simulink model "Distribution_Fault_Model"  (R2025a)
settings: Solver=VariableStepAuto  StartTime=0.0  StopTime=1  RelTol=1e-3
undefined symbols (not defined in the file or in its folder): Angle, D1, Delta, Magnitude
libraries: spsThreePhasePISectionLineLib x8, spsThreePhaseVIMeasurementLib x5, spsThreePhaseTransformerTwoWindingsLib x5, spsCurrentMeasurementLib x4, spsThreePhaseSeriesRLCLoadLib x4, spsGroundLib x3, spsVoltageMeasurementLib x3, spsThreePhaseSourceLib x1, spsThreePhaseFaultLib x1, spsSeriesRLCBranchLib x1, spspowerguiLib x1
settings Model: Creator=19092  LastModifiedBy=19092

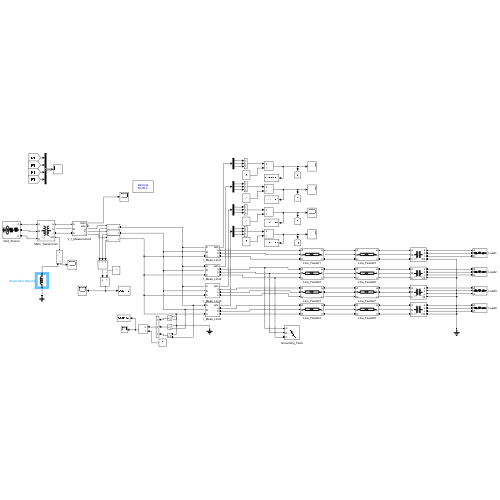
[thumbnail: Simulink's stored preview of the top-level diagram]
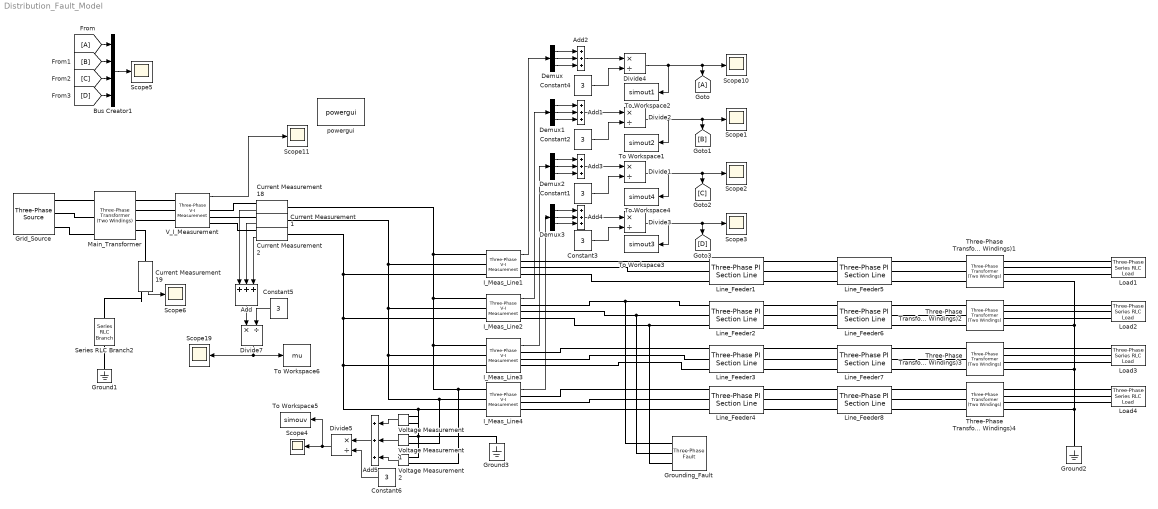
== system Distribution_Fault_Model ==
  Add{,1..5} (6 alike) : Sum  Inputs=+++
  Bus Creator1 : BusCreator  Inputs=4
  Constant{1..6} (6 alike) : Constant  Value=3
  Current Measurement{1..2,18..19} (4 alike) : spsCurrentMeasurementLib/Current Measurement  PhasorSimulation=off  OutputType=Magnitude-Angle  PSBequivalent=0
  Demux{,1..3} (4 alike) : Demux  Outputs=3
  Divide{1..5,7} (6 alike) : Product  Inputs=*/
  From : From
  Goto : Goto
  Grid_Source : spsThreePhaseSourceLib/Three-Phase Source  InternalConnection=Yg  VoltagePhases=off  Voltage=110e3  PhaseAngle=0  Voltage_phases=[25e3 25e3 25e3]/sqrt(3)  PhaseAngles_phases=[0 -120 +120]  Frequency=50  NonIdealSource=on  SpecifyImpedance=off  Resistance=0.8  Inductance=16.58e-3  ShortCircuitLevel=100e6  BaseVoltage=25e3  XRratio=7  BusType=swing  Pref=10e3  Qref=0  Prefabc=[10e3, 10e3, 10e3]  Qrefabc=[0, 0, 0]  Qmin=-inf  Qmax=inf
  Ground1 : spsGroundLib/Ground  LConnTagsString=a
  Ground2 : spsGroundLib/Ground  LConnTagsString=a
  Ground3 : spsGroundLib/Ground  LConnTagsString=a
  Grounding_Fault : spsThreePhaseFaultLib/Three-Phase Fault  InitialStates=0  FaultA=on  FaultB=off  FaultC=off  GroundFault=on  SwitchTimes=0.105  External=off  SwitchStatus=NaN  FaultResistance=100  GroundResistance=0.00000001  SnubberResistance=1e6  SnubberCapacitance=inf  Measurements=None
  I_Meas_Line{1..4} (4 alike) : spsThreePhaseVIMeasurementLib/Three-Phase V-I Measurement  VoltageMeasurement=no  SetLabelV=off  LabelV=Vabc  Vpu=off  VpuLL=off  CurrentMeasurement=yes  SetLabelI=off  LabelI=Iabc  Ipu=off  Pbase=100e6  Vbase=500e3  OutputType=Complex  PhasorSimulation=off  PSBequivalent=0
  Line_Feeder{1..4} (4 alike) : spsThreePhasePISectionLineLib/Three-Phase PI Section Line  LConnTagsString=a|b|c  RConnTagsString=A|B|C  Length=3  Frequency=50  Resistances=[0.27 2.7 ]  Inductances="[0.255e-3  1.109e-3]"  Capacitances=[0.376e-6 0.276e-6]
  Line_Feeder5 : spsThreePhasePISectionLineLib/Three-Phase PI Section Line  LConnTagsString=a|b|c  RConnTagsString=A|B|C  Length=15  Frequency=50  Resistances=[0.17 0.32 ]  Inductances="[1.017e-3  3.56e-3]"  Capacitances=[0.115e-6 0.006e-6]
  Line_Feeder6 : spsThreePhasePISectionLineLib/Three-Phase PI Section Line  LConnTagsString=a|b|c  RConnTagsString=A|B|C  Length=6  Frequency=50  Resistances=[0.27 2.7 ]  Inductances="[0.255e-3  1.109e-3]"  Capacitances=[0.376e-6 0.276e-6]
  Line_Feeder7 : spsThreePhasePISectionLineLib/Three-Phase PI Section Line  LConnTagsString=a|b|c  RConnTagsString=A|B|C  Length=6  Frequency=50  Resistances=[0.17 0.32 ]  Inductances="[ 1.017e-3  3.56e-3]"  Capacitances=[0.115e-6 0.006e-6]
  Line_Feeder8 : spsThreePhasePISectionLineLib/Three-Phase PI Section Line  LConnTagsString=a|b|c  RConnTagsString=A|B|C  Length=6  Frequency=50  Resistances=[0.17 0.32 ]  Inductances="[ 1.017e-3  3.56e-3]"  Capacitances=[0.115e-6 0.006e-6]
  Load{1..4} (4 alike) : spsThreePhaseSeriesRLCLoadLib/Three-Phase Series RLC Load  LConnTagsString=A|B|C  Configuration=Y (grounded)  NominalVoltage=380  Vabc=[1e3 1e3 1e3]  Vabcp=[1e3 1e3 1e3]  NominalFrequency=50  UnbalancedPower=off  ActivePower=0.8e5  InductivePower=0.5e5  CapacitivePower=0.2e5  Pabc=[10e3 9e3 11e3]  QLabc=[100 90 110]  QCabc=[100 90 110]  Pabcp=[10e3 9e3 11e3]  QLabcp=[100 90 110]  QCabcp=[100 90 110]  Measurements=None  LoadType=constant Z
  Main_Transformer : spsThreePhaseTransformerTwoWindingsLib/Three-Phase Transformer (Two Windings)  Winding1Connection=Yg  Winding2Connection=Yn  CoreType=Three single-phase transformers  SetSaturation=off  Hysteresis=off  DataFile='hysteresis'  SetInitialFlux=off  Measurements=None  UNITS=SI  NominalPower=[ 30e6 , 50 ]  Winding1=[1.1e+05 97.607 0.039558]  Winding2=[11000 0.0080667 3.2693e-06]  Rm=2.4402e+07  Lm=247.24  L0=0.64192  Saturation=[0 0;0.53443 343.07;222.68 434.55]  InitialFluxes=[228.71 -228.71 200.12]  BreakLoop=off  DiscreteSolver=Trapezoidal iterative  DataType=on  TransfoNumber=1
  Scope{1..6,10..11,19} (9 alike) : Scope
      Scope1 settings: ActiveDisplayYMinimum=-457.04126923383052  ActiveDisplayYMaximum=338.42605854849973  DataLoggingVariableName=ZAOlingxudianliu
      Scope10 settings: ActiveDisplayYMinimum=-5.367403011968813  ActiveDisplayYMaximum=5.1815718746200288  DataLoggingVariableName=ZAOlingxudianliu1
      Scope11 settings: ActiveDisplayYMinimum=-30411.319643702398  ActiveDisplayYMaximum=29803.514177511406
      Scope19 settings: ActiveDisplayYMinimum=-66.79577978771502  ActiveDisplayYMaximum=84.3725838120956  DataLoggingVariableName=ScopeData5
      Scope2 settings: ActiveDisplayYMinimum=-2.9181062576325916  ActiveDisplayYMaximum=2.3384047230485843  DataLoggingVariableName=ZAOlingxudianliu2
      Scope3 settings: ActiveDisplayYMinimum=-3.7719258239086075  ActiveDisplayYMaximum=3.3149529318803035  DataLoggingVariableName=ZAOlingxudianliu3
      Scope4 settings: ActiveDisplayYMinimum=-11360.33274  ActiveDisplayYMaximum=9549.66393  DataLoggingVariableName=ScopeData2
      Scope5 settings: ActiveDisplayYMinimum=-55.84943  ActiveDisplayYMaximum=52.05941
      Scope6 settings: ActiveDisplayYMinimum=-133.27899753443887  ActiveDisplayYMaximum=70.5276469261506  DataLoggingVariableName=ScopeData3
  Series RLC Branch2 : spsSeriesRLCBranchLib/Series RLC Branch  LConnTagsString=__new0  RConnTagsString=__new0  BranchType=L  Resistance=100  Inductance=0.6  SetiL0=off  InitialCurrent=0  Capacitance=1e-6  Setx0=off  InitialVoltage=0  Measurements=None
  Three-Phase Transformer (Two Windings){1..4} (4 alike) : spsThreePhaseTransformerTwoWindingsLib/Three-Phase Transformer (Two Windings)  Winding1Connection=Delta (D1)  Winding2Connection=Yn  CoreType=Three single-phase transformers  SetSaturation=off  Hysteresis=off  DataFile='hysteresis'  SetInitialFlux=off  Measurements=None  UNITS=SI  NominalPower=[5e6 , 50 ]  Winding1=[10e3 27.011 3.4392]  Winding2=[400 0.005 0.00063662]  Rm=6.7528e+06  Lm=21495  L0=0.5  Saturation=[0 0;0.10664 2292.3;44.435 2903.6]  InitialFluxes=[1528.2 -1528.2 1337.2]  BreakLoop=off  DiscreteSolver=Trapezoidal iterative  DataType=on  TransfoNumber=1
  To Workspace1 : ToWorkspace  VariableName=simout2  SaveFormat=Structure With Time  SampleTime=-1
  To Workspace2 : ToWorkspace  VariableName=simout1  SaveFormat=Structure With Time  SampleTime=-1
  To Workspace3 : ToWorkspace  VariableName=simout3  SaveFormat=Structure With Time  SampleTime=-1
  To Workspace4 : ToWorkspace  VariableName=simout4  SaveFormat=Structure With Time  SampleTime=-1
  To Workspace5 : ToWorkspace  VariableName=simouv  SaveFormat=Structure With Time  SampleTime=-1
  To Workspace6 : ToWorkspace  VariableName=mu  SaveFormat=Structure With Time  SampleTime=-1
  V_I_Measurement : spsThreePhaseVIMeasurementLib/Three-Phase V-I Measurement  VoltageMeasurement=phase-to-ground  SetLabelV=off  LabelV=Vabc  Vpu=off  VpuLL=off  CurrentMeasurement=yes  SetLabelI=off  LabelI=Iabc  Ipu=off  Pbase=100e6  Vbase=500e3  OutputType=Complex  PhasorSimulation=off  PSBequivalent=0
  Voltage Measurement : spsVoltageMeasurementLib/Voltage Measurement  PhasorSimulation=off  OutputType=Complex  PSBequivalent=0
  Voltage Measurement1 : spsVoltageMeasurementLib/Voltage Measurement  PhasorSimulation=off  OutputType=Complex  PSBequivalent=0
  Voltage Measurement2 : spsVoltageMeasurementLib/Voltage Measurement  PhasorSimulation=off  OutputType=Complex  PSBequivalent=0
  powergui : spspowerguiLib/powergui  Priority=1  SimulationMode=Discrete  SampleTime=50e-6  frequency=50  Iterations=50  frequencyindice=50  Pbase=100e6  ErrMax=1e-4  UnitsV=kV  UnitsW=MW  buscounter=0  FunctionMessages=off  echomessages=off  EnableUseOfTLC=off  CurrentSourceSwitches=off  DisableSnubberDevices=off  DisableRonSwitches=off  DisableVfSwitches=off  DisplayEquations=off  AutomaticDiscreteSolvers=off  SolverType=Tustin/Backward Euler (TBE)  Interpol=off  ExternalGateDelay=off  methode=off  Ts=100  x0status=blocks  SPID=on  SwTol=0  HookPort=off  NonlinearTolerance=1e-4  nMaxIteration=100  ContinueOnMaxIteration=off  RestoreLinks=warning  ResistiveCurrentMeasurement=off  Frange=[0:2:500]  Ylog=off  Xlog=on  ShowGrid=off  save=off  variable=ZData  structure=0  ZoomFFT=off  StartTime=0.0  cycles=1  DisplayStyle=1  fundamental=50  FreqAxis=off  MaxFrequency=1000  frequencyindicesteady=1  RmsSteady=1  display=off
  wires:
  V_I_Measurement/1 -> Scope11/1
  Current Measurement18/1 -> Add/1
  Current Measurement1/1 -> Add/2
  Current Measurement2/1 -> Add/3
  I_Meas_Line1/1 -> Demux/1
  I_Meas_Line2/1 -> Demux1/1
  I_Meas_Line4/1 -> Demux3/1
  Demux/1 -> Add2/1
  Demux/2 -> Add2/2
  Demux/3 -> Add2/3
  Demux1/1 -> Add1/1
  Demux1/2 -> Add1/2
  Demux1/3 -> Add1/3
  Demux2/1 -> Add3/1
  Demux2/2 -> Add3/2
  Demux2/3 -> Add3/3
  Demux3/1 -> Add4/1
  Demux3/2 -> Add4/2
  Demux3/3 -> Add4/3
  Add4/1 -> Divide3/1
  Constant3/1 -> Divide3/2
  Constant1/1 -> Divide1/2
  Add3/1 -> Divide1/1
  Constant2/1 -> Divide2/2
  Add1/1 -> Divide2/1
  Constant4/1 -> Divide4/2
  Add2/1 -> Divide4/1
  I_Meas_Line3/1 -> Demux2/1
  Divide3/1 -> [D], Scope3/1, To Workspace3/1
  Divide1/1 -> [C], Scope2/1, To Workspace4/1
  Divide2/1 -> [B], Scope1/1, To Workspace1/1
  Divide4/1 -> Goto/1, Scope10/1, To Workspace2/1
  [C] -> Bus Creator1/3
  [B] -> Bus Creator1/2
  From/1 -> Bus Creator1/1
  [D] -> Bus Creator1/4
  Bus Creator1/1 -> Scope5/1
  Current Measurement19/1 -> Scope6/1
  Constant5/1 -> Divide7/2
  Add/1 -> Divide7/1
  Divide7/1 -> Scope19/1, To Workspace6/1
  Constant6/1 -> Divide5/2
  Add5/1 -> Divide5/1
  Voltage Measurement/1 -> Add5/1
  Voltage Measurement1/1 -> Add5/2
  Voltage Measurement2/1 -> Add5/3
  Divide5/1 -> To Workspace5/1, Scope4/1
  connections:
  Grid_Source/RConn1 -- Main_Transformer/LConn1
  Grid_Source/RConn2 -- Main_Transformer/LConn2
  Grid_Source/RConn3 -- Main_Transformer/LConn3
  Main_Transformer/RConn1 -- V_I_Measurement/LConn1
  Main_Transformer/RConn2 -- V_I_Measurement/LConn2
  Main_Transformer/RConn3 -- V_I_Measurement/LConn3
  V_I_Measurement/RConn1 -- Current Measurement18/RConn1
  V_I_Measurement/RConn2 -- Current Measurement1/RConn1
  V_I_Measurement/RConn3 -- Current Measurement2/RConn1
  I_Meas_Line1/RConn2 -- Line_Feeder1/LConn2
  I_Meas_Line1/RConn3 -- Line_Feeder1/LConn3
  Line_Feeder1/LConn1 -- I_Meas_Line1/RConn1
  I_Meas_Line2/RConn1 -- Grounding_Fault/LConn1 -- Line_Feeder2/LConn1
  I_Meas_Line2/RConn2 -- Grounding_Fault/LConn2 -- Line_Feeder2/LConn2
  I_Meas_Line2/RConn3 -- Grounding_Fault/LConn3 -- Line_Feeder2/LConn3
  I_Meas_Line3/RConn1 -- Line_Feeder3/LConn1
  I_Meas_Line3/RConn2 -- Line_Feeder3/LConn2
  I_Meas_Line3/RConn3 -- Line_Feeder3/LConn3
  I_Meas_Line4/RConn1 -- Line_Feeder4/LConn1
  I_Meas_Line4/RConn2 -- Line_Feeder4/LConn2
  I_Meas_Line4/RConn3 -- Line_Feeder4/LConn3
  Line_Feeder5/LConn1 -- Line_Feeder1/RConn1
  Line_Feeder5/LConn2 -- Line_Feeder1/RConn2
  Line_Feeder5/LConn3 -- Line_Feeder1/RConn3
  Line_Feeder2/RConn1 -- Line_Feeder6/LConn1
  Line_Feeder6/LConn2 -- Line_Feeder2/RConn2
  Line_Feeder2/RConn3 -- Line_Feeder6/LConn3
  Line_Feeder3/RConn1 -- Line_Feeder7/LConn1
  Line_Feeder7/LConn2 -- Line_Feeder3/RConn2
  Line_Feeder3/RConn3 -- Line_Feeder7/LConn3
  Line_Feeder8/LConn1 -- Line_Feeder4/RConn1
  Line_Feeder4/RConn2 -- Line_Feeder8/LConn2
  Line_Feeder8/LConn3 -- Line_Feeder4/RConn3
  Three-Phase Transformer (Two Windings)1/LConn1 -- Line_Feeder5/RConn1
  Three-Phase Transformer (Two Windings)1/LConn2 -- Line_Feeder5/RConn2
  Three-Phase Transformer (Two Windings)1/LConn3 -- Line_Feeder5/RConn3
  Three-Phase Transformer (Two Windings)2/LConn1 -- Line_Feeder6/RConn1
  Line_Feeder6/RConn2 -- Three-Phase Transformer (Two Windings)2/LConn2
  Three-Phase Transformer (Two Windings)2/LConn3 -- Line_Feeder6/RConn3
  Line_Feeder7/RConn1 -- Three-Phase Transformer (Two Windings)3/LConn1
  Line_Feeder7/RConn2 -- Three-Phase Transformer (Two Windings)3/LConn2
  Line_Feeder7/RConn3 -- Three-Phase Transformer (Two Windings)3/LConn3
  Line_Feeder8/RConn1 -- Three-Phase Transformer (Two Windings)4/LConn1
  Line_Feeder8/RConn2 -- Three-Phase Transformer (Two Windings)4/LConn2
  Line_Feeder8/RConn3 -- Three-Phase Transformer (Two Windings)4/LConn3
  Load2/LConn1 -- Three-Phase Transformer (Two Windings)2/RConn1
  Load2/LConn2 -- Three-Phase Transformer (Two Windings)2/RConn2
  Load2/LConn3 -- Three-Phase Transformer (Two Windings)2/RConn3
  Three-Phase Transformer (Two Windings)1/RConn1 -- Load1/LConn1
  Three-Phase Transformer (Two Windings)1/RConn2 -- Load1/LConn2
  Three-Phase Transformer (Two Windings)1/RConn3 -- Load1/LConn3
  Load3/LConn1 -- Three-Phase Transformer (Two Windings)3/RConn1
  Load3/LConn2 -- Three-Phase Transformer (Two Windings)3/RConn2
  Load3/LConn3 -- Three-Phase Transformer (Two Windings)3/RConn3
  Load4/LConn1 -- Three-Phase Transformer (Two Windings)4/RConn1
  Load4/LConn2 -- Three-Phase Transformer (Two Windings)4/RConn2
  Load4/LConn3 -- Three-Phase Transformer (Two Windings)4/RConn3
  Three-Phase Transformer (Two Windings)1/RConn4 -- Three-Phase Transformer (Two Windings)2/RConn4 -- Three-Phase Transformer (Two Windings)3/RConn4 -- Ground2/LConn1 -- Three-Phase Transformer (Two Windings)4/RConn4
  Current Measurement18/LConn1 -- I_Meas_Line1/LConn1 -- I_Meas_Line2/LConn1 -- I_Meas_Line3/LConn1 -- Voltage Measurement2/LConn1 -- I_Meas_Line4/LConn1
  Current Measurement1/LConn1 -- I_Meas_Line1/LConn2 -- I_Meas_Line2/LConn2 -- I_Meas_Line3/LConn2 -- Voltage Measurement1/LConn1 -- I_Meas_Line4/LConn2
  Current Measurement2/LConn1 -- I_Meas_Line1/LConn3 -- I_Meas_Line2/LConn3 -- I_Meas_Line3/LConn3 -- Voltage Measurement/LConn1 -- I_Meas_Line4/LConn3
  Main_Transformer/RConn4 -- Current Measurement19/LConn1
  Current Measurement19/RConn1 -- Series RLC Branch2/LConn1
  Ground1/LConn1 -- Series RLC Branch2/RConn1
  Voltage Measurement/LConn2 -- Ground3/LConn1 -- Voltage Measurement2/LConn2 -- Voltage Measurement1/LConn2
